simulink model "mrefrobotarm_modified_previous_y_previous_ref"  (R2018b)
settings: Solver=FixedStepAuto  StartTime=0.0  StopTime=60  RelTol=1e-3  AbsTol=1e-6
undefined symbols (not defined in the file or in its folder): sfunxy2
libraries: neural x301, simulink x1
(part 7 of 10)

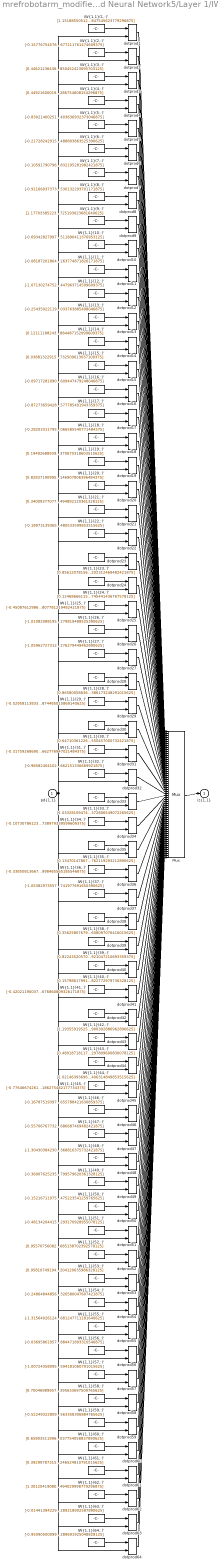
== system mrefrobotarm_modified_previous_y_previous_ref/Feed-Forward Neural Network5/Layer 1/IW{1,1} ==
  "pd{1,1}" : Inport  PortDimensions=8
      mask Display: e = 0.06;c1 = [120 230 180]/255;c2 = ([120 230 180]+0)/(256+128);c3 = ([120 230 180]+128)/(256+128);patch([0 1 1 0],[0 0 1 1],c1);patch([0 1 1 1-e 1-e 0+e],[0 0 1 1-e 0+e 0+e],c2);patch([0 0 1 1-e 0+e 0+e],[0 1 1 1-e 1-e 0+e],c3);plot([0 1 1 0 0],[0 0 1 1 0]);
  "IW{1,1}(1,:)'" : Constant  Value=[1.15188550512719078966483721160329878330230712890625;0.28812102779775983218968349319766275584697723388671875;0.56266210788343784532372637841035611927509307861328125;-0.28333109295564262719580028715427033603191375732421875;0.2157034015099435764195590081726550124585628509521484375;-0.320690714134774623733648013512720353901386260986328125;-1.7558165749549512479887880544993095099925994873046875;-0.445441972828221455227293290590750984847545623779296875]
      mask Display: e = 0.06;c1 = [120 150 230]/255;c2 = ([120 150 230]+0)/383;c3 = ([120 150 230]+128)/383;patch([0 1 1 0],[0 0 1 1],c1);patch([0 1 1 1-e 1-e 0+e],[0 0 1 1-e 0+e 0+e],c2);patch([0 0 1 1-e 0+e 0+e],[0 1 1 1-e 1-e 0+e],c3);plot([0 1 1 0 0],[0 0 1 1 0]);disp('Weights');
  "IW{1,1}(10,:)'" : Constant  Value=[-0.69342827997867140243926087350700981914997100830078125;0.302628053808435326654802111079334281384944915771484375;0.50475756804391236354234706595889292657375335693359375;-0.8382169307464308882771319986204616725444793701171875;0.514118176756543032723811847972683608531951904296875;0.9119975746533526272941116985748521983623504638671875;0.59957744726285355785222463964601047337055206298828125;0.75864381905745237322236107502249069511890411376953125]
      mask Display: e = 0.06;c1 = [120 150 230]/255;c2 = ([120 150 230]+0)/383;c3 = ([120 150 230]+128)/383;patch([0 1 1 0],[0 0 1 1],c1);patch([0 1 1 1-e 1-e 0+e],[0 0 1 1-e 0+e 0+e],c2);patch([0 0 1 1-e 0+e 0+e],[0 1 1 1-e 1-e 0+e],c3);plot([0 1 1 0 0],[0 0 1 1 0]);disp('Weights');
  "IW{1,1}(11,:)'" : Constant  Value=[-0.08187201864334088530217314882975188083946704864501953125;0.73089752966811116774437095955363474786281585693359375;0.5387200520871704423342407608288340270519256591796875;-1.09121606557834116557614834164269268512725830078125;0.9840256530079540819855310473940335214138031005859375;0.413862403720223703817993055054103024303913116455078125;1.027219477112980339228442971943877637386322021484375;-0.66505920483041236490606706865946762263774871826171875]
      mask Display: e = 0.06;c1 = [120 150 230]/255;c2 = ([120 150 230]+0)/383;c3 = ([120 150 230]+128)/383;patch([0 1 1 0],[0 0 1 1],c1);patch([0 1 1 1-e 1-e 0+e],[0 0 1 1-e 0+e 0+e],c2);patch([0 0 1 1-e 0+e 0+e],[0 1 1 1-e 1-e 0+e],c3);plot([0 1 1 0 0],[0 0 1 1 0]);disp('Weights');
  "IW{1,1}(12,:)'" : Constant  Value=[-1.07130274752541776450698307598941028118133544921875;-1.4362522873395537903462582107749767601490020751953125;0.32170080578624327127812421167618595063686370849609375;1.03829812140938404496637303964234888553619384765625;-0.759812891496933762169874171377159655094146728515625;0.602197452374559016874400185770355165004730224609375;0.2151555708852344872550332866012468002736568450927734375;0.328318123712607989883593972990638576447963714599609375]
      mask Display: e = 0.06;c1 = [120 150 230]/255;c2 = ([120 150 230]+0)/383;c3 = ([120 150 230]+128)/383;patch([0 1 1 0],[0 0 1 1],c1);patch([0 1 1 1-e 1-e 0+e],[0 0 1 1-e 0+e 0+e],c2);patch([0 0 1 1-e 0+e 0+e],[0 1 1 1-e 1-e 0+e],c3);plot([0 1 1 0 0],[0 0 1 1 0]);disp('Weights');
  "IW{1,1}(13,:)'" : Constant  Value=[-0.254350221196234016485249185279826633632183074951171875;-1.1795238596441508516221574609517119824886322021484375;0.80833668204856368166844049483188427984714508056640625;0.86038083232116691068114278095890767872333526611328125;-0.450732077477428216827348705919575877487659454345703125;-1.0998838119882419217532287802896462380886077880859375;0.50040120768586004995626126401475630700588226318359375;-0.780004345720864744606615204247646033763885498046875]
      mask Display: e = 0.06;c1 = [120 150 230]/255;c2 = ([120 150 230]+0)/383;c3 = ([120 150 230]+128)/383;patch([0 1 1 0],[0 0 1 1],c1);patch([0 1 1 1-e 1-e 0+e],[0 0 1 1-e 0+e 0+e],c2);patch([0 0 1 1-e 0+e 0+e],[0 1 1 1-e 1-e 0+e],c3);plot([0 1 1 0 0],[0 0 1 1 0]);disp('Weights');
  "IW{1,1}(14,:)'" : Constant  Value=[0.12111188243225030902738836857679416425526142120361328125;1.2254734338665216331065721533377654850482940673828125;-1.2126460475572156116896849198383279144763946533203125;-0.11392876827753649349173059590611956082284450531005859375;0.1615772181693192199869457681415951810777187347412109375;1.061583549738458032152266241610050201416015625;0.10245837646828574729607197468794765882194042205810546875;1.14489655514380839207433382398448884487152099609375]
      mask Display: e = 0.06;c1 = [120 150 230]/255;c2 = ([120 150 230]+0)/383;c3 = ([120 150 230]+128)/383;patch([0 1 1 0],[0 0 1 1],c1);patch([0 1 1 1-e 1-e 0+e],[0 0 1 1-e 0+e 0+e],c2);patch([0 0 1 1-e 0+e 0+e],[0 1 1 1-e 1-e 0+e],c3);plot([0 1 1 0 0],[0 0 1 1 0]);disp('Weights');
  "IW{1,1}(15,:)'" : Constant  Value=[0.038813229156217245174875785096446634270250797271728515625;0.486470279353224788199128170163021422922611236572265625;-0.45894295845177135451109506902866996824741363525390625;0.0276916856546326091426113436000377987511456012725830078125;1.6051967623725589273675495860516093671321868896484375;-0.45590732770331587886403212905861437320709228515625;-0.652539724709438218042123480699956417083740234375;1.0980322803721804802989936433732509613037109375]
      mask Display: e = 0.06;c1 = [120 150 230]/255;c2 = ([120 150 230]+0)/383;c3 = ([120 150 230]+128)/383;patch([0 1 1 0],[0 0 1 1],c1);patch([0 1 1 1-e 1-e 0+e],[0 0 1 1-e 0+e 0+e],c2);patch([0 0 1 1-e 0+e 0+e],[0 1 1 1-e 1-e 0+e],c3);plot([0 1 1 0 0],[0 0 1 1 0]);disp('Weights');
  "IW{1,1}(16,:)'" : Constant  Value=[-0.097172810908892959247395992861129343509674072265625;1.21828113992966802214823474059812724590301513671875;-0.348946678645212615688109281109063886106014251708984375;1.6228867623269358499982217836077325046062469482421875;-0.4468755805697319782865406523342244327068328857421875;0.25552428628844126023977878503501415252685546875;-0.841604705929505758632558354292996227741241455078125;0.384149848353079359508654988530906848609447479248046875]
      mask Display: e = 0.06;c1 = [120 150 230]/255;c2 = ([120 150 230]+0)/383;c3 = ([120 150 230]+128)/383;patch([0 1 1 0],[0 0 1 1],c1);patch([0 1 1 1-e 1-e 0+e],[0 0 1 1-e 0+e 0+e],c2);patch([0 0 1 1-e 0+e 0+e],[0 1 1 1-e 1-e 0+e],c3);plot([0 1 1 0 0],[0 0 1 1 0]);disp('Weights');
  "IW{1,1}(17,:)'" : Constant  Value=[-0.8727365942863782866112387637258507311344146728515625;-1.126434571242459714568440176662988960742950439453125;0.36545685371113723061142763981479220092296600341796875;0.962011466852533470017760919290594756603240966796875;-0.68899715378819259559151078065042383968830108642578125;-0.59210547871686614040953600124339573085308074951171875;-0.06602088688853786913046661766202305443584918975830078125;1.1033314028657768002261718720546923577785491943359375]
      mask Display: e = 0.06;c1 = [120 150 230]/255;c2 = ([120 150 230]+0)/383;c3 = ([120 150 230]+128)/383;patch([0 1 1 0],[0 0 1 1],c1);patch([0 1 1 1-e 1-e 0+e],[0 0 1 1-e 0+e 0+e],c2);patch([0 0 1 1-e 0+e 0+e],[0 1 1 1-e 1-e 0+e],c3);plot([0 1 1 0 0],[0 0 1 1 0]);disp('Weights');
  "IW{1,1}(18,:)'" : Constant  Value=[-0.282033117955742096416571484951418824493885040283203125;-0.09685575267191497139673828087325091473758220672607421875;1.0369904994954521892935872529051266610622406005859375;0.410108416989715340861266668071039021015167236328125;0.5329483580200420345107659159111790359020233154296875;1.0824307275914344383949128314270637929439544677734375;1.0907238106762771057134386865072883665561676025390625;-0.9864564974524812068779056062339805066585540771484375]
      mask Display: e = 0.06;c1 = [120 150 230]/255;c2 = ([120 150 230]+0)/383;c3 = ([120 150 230]+128)/383;patch([0 1 1 0],[0 0 1 1],c1);patch([0 1 1 1-e 1-e 0+e],[0 0 1 1-e 0+e 0+e],c2);patch([0 0 1 1-e 0+e 0+e],[0 1 1 1-e 1-e 0+e],c3);plot([0 1 1 0 0],[0 0 1 1 0]);disp('Weights');
  "IW{1,1}(19,:)'" : Constant  Value=[0.19492688939710911544267446515732444822788238525390625;0.28850729483225101557053449141676537692546844482421875;-0.175773740393380395463651666432269848883152008056640625;-1.89756443554498854808798569138161838054656982421875;-0.5054315086265079859373372528352774679660797119140625;1.0667368662509619792189141662674956023693084716796875;0.19891400645817736148046606103889644145965576171875;0.567362684381534254640655490220524370670318603515625]
      mask Display: e = 0.06;c1 = [120 150 230]/255;c2 = ([120 150 230]+0)/383;c3 = ([120 150 230]+128)/383;patch([0 1 1 0],[0 0 1 1],c1);patch([0 1 1 1-e 1-e 0+e],[0 0 1 1-e 0+e 0+e],c2);patch([0 0 1 1-e 0+e 0+e],[0 1 1 1-e 1-e 0+e],c3);plot([0 1 1 0 0],[0 0 1 1 0]);disp('Weights');
  "IW{1,1}(2,:)'" : Constant  Value=[-0.15776754576942597640965004757163114845752716064453125;-0.455993213383465434418440054287202656269073486328125;1.1839932390166734155201311295968480408191680908203125;0.29937087607287893309404580577393062412738800048828125;-0.0048999116352581063849047637859257520176470279693603515625;0.049281318949005371854443779966459260322153568267822265625;-1.1301308079633043401912573244771920144557952880859375;-1.494209820076525030430047991103492677211761474609375]
      mask Display: e = 0.06;c1 = [120 150 230]/255;c2 = ([120 150 230]+0)/383;c3 = ([120 150 230]+128)/383;patch([0 1 1 0],[0 0 1 1],c1);patch([0 1 1 1-e 1-e 0+e],[0 0 1 1-e 0+e 0+e],c2);patch([0 0 1 1-e 0+e 0+e],[0 1 1 1-e 1-e 0+e],c3);plot([0 1 1 0 0],[0 0 1 1 0]);disp('Weights');
  "IW{1,1}(20,:)'" : Constant  Value=[0.8283719099560700183104700045078061521053314208984375;-0.9420385849900030361681046997546218335628509521484375;0.83950886137076008441937347015482373535633087158203125;-0.94073002472129407802725609144545160233974456787109375;-0.58905367954073117875424259182182140648365020751953125;0.9613658421825383992853630843455903232097625732421875;0.6352455319925611743059334912686608731746673583984375;0.551159922915347433303168145357631146907806396484375]
      mask Display: e = 0.06;c1 = [120 150 230]/255;c2 = ([120 150 230]+0)/383;c3 = ([120 150 230]+128)/383;patch([0 1 1 0],[0 0 1 1],c1);patch([0 1 1 1-e 1-e 0+e],[0 0 1 1-e 0+e 0+e],c2);patch([0 0 1 1-e 0+e 0+e],[0 1 1 1-e 1-e 0+e],c3);plot([0 1 1 0 0],[0 0 1 1 0]);disp('Weights');
  "IW{1,1}(21,:)'" : Constant  Value=[0.34009377077838232050766009706421755254268646240234375;-0.466780497991363285681387651493423618376255035400390625;1.2292709966424573142518283930257894098758697509765625;-0.88137293354350243479444770855479873716831207275390625;-0.7761093614509670945977859446429647505283355712890625;-0.160844472776546176806533594572101719677448272705078125;0.9128574666560584915941944927908480167388916015625;-1.0472251078619354558441045810468494892120361328125]
      mask Display: e = 0.06;c1 = [120 150 230]/255;c2 = ([120 150 230]+0)/383;c3 = ([120 150 230]+128)/383;patch([0 1 1 0],[0 0 1 1],c1);patch([0 1 1 1-e 1-e 0+e],[0 0 1 1-e 0+e 0+e],c2);patch([0 0 1 1-e 0+e 0+e],[0 1 1 1-e 1-e 0+e],c3);plot([0 1 1 0 0],[0 0 1 1 0]);disp('Weights');
  "IW{1,1}(22,:)'" : Constant  Value=[-0.189731393651665081190316186621203087270259857177734375;-0.72495794035112359754435829017893411219120025634765625;0.9357984514248178786743892487720586359500885009765625;-1.0869305870717254070001445143134333193302154541015625;-0.50973886964233405816315780612058006227016448974609375;0.473915859680547002508177456547855399549007415771484375;1.0230173709565664186271760627278126776218414306640625;0.9914709747258270144953939961851574480533599853515625]
      mask Display: e = 0.06;c1 = [120 150 230]/255;c2 = ([120 150 230]+0)/383;c3 = ([120 150 230]+128)/383;patch([0 1 1 0],[0 0 1 1],c1);patch([0 1 1 1-e 1-e 0+e],[0 0 1 1-e 0+e 0+e],c2);patch([0 0 1 1-e 0+e 0+e],[0 1 1 1-e 1-e 0+e],c3);plot([0 1 1 0 0],[0 0 1 1 0]);disp('Weights');
  "IW{1,1}(23,:)'" : Constant  Value=[0.856120781560206989269090627203695476055145263671875;-1.069464124720405973079095929278992116451263427734375;0.2919731447302797988641032134182751178741455078125;0.6061622306072764754247828022926114499568939208984375;-0.653691930601032478165279826498590409755706787109375;-0.88804792534942789128393769715330563485622406005859375;-1.0119635839619267603239904929068870842456817626953125;0.95988282102991540067904452371294610202312469482421875]
      mask Display: e = 0.06;c1 = [120 150 230]/255;c2 = ([120 150 230]+0)/383;c3 = ([120 150 230]+128)/383;patch([0 1 1 0],[0 0 1 1],c1);patch([0 1 1 1-e 1-e 0+e],[0 0 1 1-e 0+e 0+e],c2);patch([0 0 1 1-e 0+e 0+e],[0 1 1 1-e 1-e 0+e],c3);plot([0 1 1 0 0],[0 0 1 1 0]);disp('Weights');
  "IW{1,1}(24,:)'" : Constant  Value=[0.124686661157710043656976495185517705976963043212890625;-0.8210810741082565922255298573873005807399749755859375;1.1767856627094956945001058556954376399517059326171875;0.1691193234330329586700969457524479366838932037353515625;-1.12605095295487611650742110214196145534515380859375;-0.96214809238136800306762097534374333918094635009765625;-0.95747311663602430176212010337621904909610748291015625;-0.8403367277084676789655759421293623745441436767578125]
      mask Display: e = 0.06;c1 = [120 150 230]/255;c2 = ([120 150 230]+0)/383;c3 = ([120 150 230]+128)/383;patch([0 1 1 0],[0 0 1 1],c1);patch([0 1 1 1-e 1-e 0+e],[0 0 1 1-e 0+e 0+e],c2);patch([0 0 1 1-e 0+e 0+e],[0 1 1 1-e 1-e 0+e],c3);plot([0 1 1 0 0],[0 0 1 1 0]);disp('Weights');
  "IW{1,1}(25,:)'" : Constant  Value=[-0.4508761298608821022071424522437155246734619140625;1.0106688771579630525820903130806982517242431640625;-0.1774785669335633697674126096899271942675113677978515625;0.488867822831043519204996528060291893780231475830078125;-0.523769084982353749779804275021888315677642822265625;0.5469050128236101482315234534326009452342987060546875;1.628688158073976932627147107268683612346649169921875;0.2267927559895878963924786830830271355807781219482421875]
      mask Display: e = 0.06;c1 = [120 150 230]/255;c2 = ([120 150 230]+0)/383;c3 = ([120 150 230]+128)/383;patch([0 1 1 0],[0 0 1 1],c1);patch([0 1 1 1-e 1-e 0+e],[0 0 1 1-e 0+e 0+e],c2);patch([0 0 1 1-e 0+e 0+e],[0 1 1 1-e 1-e 0+e],c3);plot([0 1 1 0 0],[0 0 1 1 0]);disp('Weights');
  "IW{1,1}(26,:)'" : Constant  Value=[-1.01082088195786301554335295804776251316070556640625;0.95465379283400275678417301605804823338985443115234375;0.391386386609228142940963834917056374251842498779296875;1.4225990849750778100002435166970826685428619384765625;-0.73545495103985902840548760650563053786754608154296875;-0.736133991802305320817367828567512333393096923828125;0.442114848390933234956179376240470446646213531494140625;0.43657172644220987312024817583733238279819488525390625]
      mask Display: e = 0.06;c1 = [120 150 230]/255;c2 = ([120 150 230]+0)/383;c3 = ([120 150 230]+128)/383;patch([0 1 1 0],[0 0 1 1],c1);patch([0 1 1 1-e 1-e 0+e],[0 0 1 1-e 0+e 0+e],c2);patch([0 0 1 1-e 0+e 0+e],[0 1 1 1-e 1-e 0+e],c3);plot([0 1 1 0 0],[0 0 1 1 0]);disp('Weights');
  "IW{1,1}(27,:)'" : Constant  Value=[-1.0596272731227285301969232023111544549465179443359375;-0.54530840839943228726127699701464734971523284912109375;0.6278313816556941873159303213469684123992919921875;0.270771156859894279733680377830751240253448486328125;0.464390599696782147010054586644400842487812042236328125;-0.53372241047857371665230630242149345576763153076171875;0.956306487503788549275896002654917538166046142578125;1.47074764980775629652498537325300276279449462890625]
      mask Display: e = 0.06;c1 = [120 150 230]/255;c2 = ([120 150 230]+0)/383;c3 = ([120 150 230]+128)/383;patch([0 1 1 0],[0 0 1 1],c1);patch([0 1 1 1-e 1-e 0+e],[0 0 1 1-e 0+e 0+e],c2);patch([0 0 1 1-e 0+e 0+e],[0 1 1 1-e 1-e 0+e],c3);plot([0 1 1 0 0],[0 0 1 1 0]);disp('Weights');
  "IW{1,1}(28,:)'" : Constant  Value=[0.86580058636540346839183257543481886386871337890625;0.9756419600736609964997114730067551136016845703125;-1.2316073907028701750476784582133404910564422607421875;-1.03033429662976772078764042817056179046630859375;0.1339502814816569686851011056205607019364833831787109375;0.74929830934803554054468577305669896304607391357421875;0.0743680662885670973327734145641443319618701934814453125;-0.80516734717865345860587922288686968386173248291015625]
      mask Display: e = 0.06;c1 = [120 150 230]/255;c2 = ([120 150 230]+0)/383;c3 = ([120 150 230]+128)/383;patch([0 1 1 0],[0 0 1 1],c1);patch([0 1 1 1-e 1-e 0+e],[0 0 1 1-e 0+e 0+e],c2);patch([0 0 1 1-e 0+e 0+e],[0 1 1 1-e 1-e 0+e],c3);plot([0 1 1 0 0],[0 0 1 1 0]);disp('Weights');
  "IW{1,1}(29,:)'" : Constant  Value=[-0.5295811383351869405800016465946100652217864990234375;-0.278717330509984650976917919251718558371067047119140625;-0.66606714661326493764903489136486314237117767333984375;-0.8798401281044869737257840824895538389682769775390625;0.268788230217950785405633951086201705038547515869140625;-1.5135879192232033485510100945248268544673919677734375;0.91318255242783175074094970113947056233882904052734375;0.920699349371988606804961818852461874485015869140625]
      mask Display: e = 0.06;c1 = [120 150 230]/255;c2 = ([120 150 230]+0)/383;c3 = ([120 150 230]+128)/383;patch([0 1 1 0],[0 0 1 1],c1);patch([0 1 1 1-e 1-e 0+e],[0 0 1 1-e 0+e 0+e],c2);patch([0 0 1 1-e 0+e 0+e],[0 1 1 1-e 1-e 0+e],c3);plot([0 1 1 0 0],[0 0 1 1 0]);disp('Weights');
  "IW{1,1}(3,:)'" : Constant  Value=[0.446212364360280389075086304728756658732891082763671875;-0.0978189681976021907505725039300159551203250885009765625;-1.31393838489276415515405460610054433345794677734375;-0.79167290442859183929869004714419133961200714111328125;1.1377022565084218275188732150127179920673370361328125;0.0090609210361883817108630267966873361729085445404052734375;-1.231014577077934379900625572190620005130767822265625;-0.1951198768884519207933436746316147036850452423095703125]
      mask Display: e = 0.06;c1 = [120 150 230]/255;c2 = ([120 150 230]+0)/383;c3 = ([120 150 230]+128)/383;patch([0 1 1 0],[0 0 1 1],c1);patch([0 1 1 1-e 1-e 0+e],[0 0 1 1-e 0+e 0+e],c2);patch([0 0 1 1-e 0+e 0+e],[0 1 1 1-e 1-e 0+e],c3);plot([0 1 1 0 0],[0 0 1 1 0]);disp('Weights');
  "IW{1,1}(30,:)'" : Constant  Value=[0.6471036122667062073787747067399322986602783203125;-0.061940615906763842046789392270511598326265811920166015625;-0.312052580594836259653135357439168728888034820556640625;1.2990947753306822942676035381737165153026580810546875;-0.0036105482406158756307490431680662368307821452617645263671875;-0.42311702194302835966510656362515874207019805908203125;0.88830861509092995387248947736225090920925140380859375;-1.6478565407139675880188178780372254550457000732421875]
      mask Display: e = 0.06;c1 = [120 150 230]/255;c2 = ([120 150 230]+0)/383;c3 = ([120 150 230]+128)/383;patch([0 1 1 0],[0 0 1 1],c1);patch([0 1 1 1-e 1-e 0+e],[0 0 1 1-e 0+e 0+e],c2);patch([0 0 1 1-e 0+e 0+e],[0 1 1 1-e 1-e 0+e],c3);plot([0 1 1 0 0],[0 0 1 1 0]);disp('Weights');
  "IW{1,1}(31,:)'" : Constant  Value=[-0.31759268690855346761736655025742948055267333984375;-0.4042457377349506497665743154357187449932098388671875;0.251357110918958459588878895374364219605922698974609375;-1.10791367956164332753132839570753276348114013671875;0.73836626855680165260054081954876892268657684326171875;1.032559094167967206345792874344624578952789306640625;-1.070606342674453426155878332792781293392181396484375;1.126008088640405357949703102349303662776947021484375]
      mask Display: e = 0.06;c1 = [120 150 230]/255;c2 = ([120 150 230]+0)/383;c3 = ([120 150 230]+128)/383;patch([0 1 1 0],[0 0 1 1],c1);patch([0 1 1 1-e 1-e 0+e],[0 0 1 1-e 0+e 0+e],c2);patch([0 0 1 1-e 0+e 0+e],[0 1 1 1-e 1-e 0+e],c3);plot([0 1 1 0 0],[0 0 1 1 0]);disp('Weights');
  "IW{1,1}(32,:)'" : Constant  Value=[-0.98582404102823650848819170278147794306278228759765625;0.110955204356297743029102775835781358182430267333984375;1.1171545662955260080906327857519499957561492919921875;-0.086582673998257642100639941418194212019443511962890625;1.0183086056376919881216736030182801187038421630859375;-0.146176428296484084423667582086636684834957122802734375;-1.27212378176424056874793677707202732563018798828125;0.778085451655250448510514615918509662151336669921875]
      mask Display: e = 0.06;c1 = [120 150 230]/255;c2 = ([120 150 230]+0)/383;c3 = ([120 150 230]+128)/383;patch([0 1 1 0],[0 0 1 1],c1);patch([0 1 1 1-e 1-e 0+e],[0 0 1 1-e 0+e 0+e],c2);patch([0 0 1 1-e 0+e 0+e],[0 1 1 1-e 1-e 0+e],c3);plot([0 1 1 0 0],[0 0 1 1 0]);disp('Weights');
  "IW{1,1}(33,:)'" : Constant  Value=[1.0332810947416766200745996684418059885501861572265625;1.1881751882562401334553214837796986103057861328125;0.0113711764073888312032156733266674564220011234283447265625;0.54613530436783752630702792885131202638149261474609375;0.8575124714924264868187719912384636700153350830078125;-0.9807149901858362994744311436079442501068115234375;-0.08504032072985522050512230407548486255109310150146484375;-0.86010602226781662782428838909254409372806549072265625]
      mask Display: e = 0.06;c1 = [120 150 230]/255;c2 = ([120 150 230]+0)/383;c3 = ([120 150 230]+128)/383;patch([0 1 1 0],[0 0 1 1],c1);patch([0 1 1 1-e 1-e 0+e],[0 0 1 1-e 0+e 0+e],c2);patch([0 0 1 1-e 0+e 0+e],[0 1 1 1-e 1-e 0+e],c3);plot([0 1 1 0 0],[0 0 1 1 0]);disp('Weights');
  "IW{1,1}(34,:)'" : Constant  Value=[-0.10730786123257247954843052184514817781746387481689453125;-1.2561740133845915590171671283314935863018035888671875;0.1916023081249165205264262112905271351337432861328125;-0.733724466418752552243631726014427840709686279296875;-1.19798795607447328137595832231454551219940185546875;0.395299789476157126255628782018902711570262908935546875;1.2942966424689743565323851726134307682514190673828125;0.2851043720773309697591457734233699738979339599609375]
      mask Display: e = 0.06;c1 = [120 150 230]/255;c2 = ([120 150 230]+0)/383;c3 = ([120 150 230]+128)/383;patch([0 1 1 0],[0 0 1 1],c1);patch([0 1 1 1-e 1-e 0+e],[0 0 1 1-e 0+e 0+e],c2);patch([0 0 1 1-e 0+e 0+e],[0 1 1 1-e 1-e 0+e],c3);plot([0 1 1 0 0],[0 0 1 1 0]);disp('Weights');
  "IW{1,1}(35,:)'" : Constant  Value=[0.13470147867077508774258376433863304555416107177734375;0.89180318892628818172596538715879432857036590576171875;-1.251923878018734281880597336567007005214691162109375;1.0584028339053215272969055149587802588939666748046875;-0.466690066426573457736282080077216960489749908447265625;0.80408658190793047548794447720865719020366668701171875;0.80069797512159424091038317783386446535587310791015625;0.65001316148328280863921690979623235762119293212890625]
      mask Display: e = 0.06;c1 = [120 150 230]/255;c2 = ([120 150 230]+0)/383;c3 = ([120 150 230]+128)/383;patch([0 1 1 0],[0 0 1 1],c1);patch([0 1 1 1-e 1-e 0+e],[0 0 1 1-e 0+e 0+e],c2);patch([0 0 1 1-e 0+e 0+e],[0 1 1 1-e 1-e 0+e],c3);plot([0 1 1 0 0],[0 0 1 1 0]);disp('Weights');
  "IW{1,1}(36,:)'" : Constant  Value=[-0.3385081366785949175124414978199638426303863525390625;-0.69503528690295102165919161052443087100982666015625;0.4923281094682134817475116506102494895458221435546875;-0.720964622145814804099472894449718296527862548828125;-0.2556243474584316555109353430452756583690643310546875;-1.1219523070902417405392270666197873651981353759765625;-1.060868790922331328374639269895851612091064453125;-1.28292959603458012196597337606362998485565185546875]
      mask Display: e = 0.06;c1 = [120 150 230]/255;c2 = ([120 150 230]+0)/383;c3 = ([120 150 230]+128)/383;patch([0 1 1 0],[0 0 1 1],c1);patch([0 1 1 1-e 1-e 0+e],[0 0 1 1-e 0+e 0+e],c2);patch([0 0 1 1-e 0+e 0+e],[0 1 1 1-e 1-e 0+e],c3);plot([0 1 1 0 0],[0 0 1 1 0]);disp('Weights');
  "IW{1,1}(37,:)'" : Constant  Value=[-1.0538297355717778369665893478668294847011566162109375;0.9137438889102564854027832552674226462841033935546875;0.330465292020934608974158663841080851852893829345703125;-0.469046635263795697046163013510522432625293731689453125;0.76983143635499262646959550693281926214694976806640625;1.2274381452821707672029560853843577206134796142578125;-0.9594647793827260073840079712681472301483154296875;0.4807491192598087881293622558587230741977691650390625]
      mask Display: e = 0.06;c1 = [120 150 230]/255;c2 = ([120 150 230]+0)/383;c3 = ([120 150 230]+128)/383;patch([0 1 1 0],[0 0 1 1],c1);patch([0 1 1 1-e 1-e 0+e],[0 0 1 1-e 0+e 0+e],c2);patch([0 0 1 1-e 0+e 0+e],[0 1 1 1-e 1-e 0+e],c3);plot([0 1 1 0 0],[0 0 1 1 0]);disp('Weights');
  "IW{1,1}(38,:)'" : Constant  Value=[0.35625807679689269757972169827553443610668182373046875;0.1331977864564148072989979709745966829359531402587890625;-0.365682952283444662189282325925887562334537506103515625;-1.0953170441072181962027798363124020397663116455078125;0.8305354135097473555759961527655832469463348388671875;1.085738228001417837731423787772655487060546875;1.0659017284151206528264310691156424582004547119140625;0.807218132587677050793217858881689608097076416015625]
      mask Display: e = 0.06;c1 = [120 150 230]/255;c2 = ([120 150 230]+0)/383;c3 = ([120 150 230]+128)/383;patch([0 1 1 0],[0 0 1 1],c1);patch([0 1 1 1-e 1-e 0+e],[0 0 1 1-e 0+e 0+e],c2);patch([0 0 1 1-e 0+e 0+e],[0 1 1 1-e 1-e 0+e],c3);plot([0 1 1 0 0],[0 0 1 1 0]);disp('Weights');
  "IW{1,1}(39,:)'" : Constant  Value=[0.82243520570661321489325246147927828133106231689453125;-0.92744873138334449347297550048097036778926849365234375;-0.5659382507761587799421931777033023536205291748046875;1.10287668857012288725627513485960662364959716796875;0.6500558112044181324762348594958893954753875732421875;-0.279365585293477491912739196777692995965480804443359375;-0.329420056930422811003467131740762852132320404052734375;1.214469321330822193516496554366312921047210693359375]
      mask Display: e = 0.06;c1 = [120 150 230]/255;c2 = ([120 150 230]+0)/383;c3 = ([120 150 230]+128)/383;patch([0 1 1 0],[0 0 1 1],c1);patch([0 1 1 1-e 1-e 0+e],[0 0 1 1-e 0+e 0+e],c2);patch([0 0 1 1-e 0+e 0+e],[0 1 1 1-e 1-e 0+e],c3);plot([0 1 1 0 0],[0 0 1 1 0]);disp('Weights');
  "IW{1,1}(4,:)'" : Constant  Value=[0.449216000193385534000611869487329386174678802490234375;1.069092416755129004712898677098564803600311279296875;1.1202529630482478406605650889105163514614105224609375;0.88723055542406170648206398254842497408390045166015625;-0.53693856516414084634192249723128043115139007568359375;-0.8953535921229356375761199160479009151458740234375;-0.424853262852135316052226698957383632659912109375;0.98558770378236093545609719512867741286754608154296875]
      mask Display: e = 0.06;c1 = [120 150 230]/255;c2 = ([120 150 230]+0)/383;c3 = ([120 150 230]+128)/383;patch([0 1 1 0],[0 0 1 1],c1);patch([0 1 1 1-e 1-e 0+e],[0 0 1 1-e 0+e 0+e],c2);patch([0 0 1 1-e 0+e 0+e],[0 1 1 1-e 1-e 0+e],c3);plot([0 1 1 0 0],[0 0 1 1 0]);disp('Weights');
  "IW{1,1}(40,:)'" : Constant  Value=[0.1579861799126709431817516815499402582645416259765625;0.2440200417363912188672969705294235609471797943115234375;-1.254796483799876849474230766645632684230804443359375;0.5053076788989432355236885996419005095958709716796875;0.050687802700905726371871651281253434717655181884765625;1.485676910567629960269186994992196559906005859375;-0.4868889044458868387010852529783733189105987548828125;0.86657970142906493027368242110242135822772979736328125]
      mask Display: e = 0.06;c1 = [120 150 230]/255;c2 = ([120 150 230]+0)/383;c3 = ([120 150 230]+128)/383;patch([0 1 1 0],[0 0 1 1],c1);patch([0 1 1 1-e 1-e 0+e],[0 0 1 1-e 0+e 0+e],c2);patch([0 0 1 1-e 0+e 0+e],[0 1 1 1-e 1-e 0+e],c3);plot([0 1 1 0 0],[0 0 1 1 0]);disp('Weights');
  "IW{1,1}(41,:)'" : Constant  Value=[-0.420211900371094182471409794743522070348262786865234375;-0.27063223612642517412751885785837657749652862548828125;-1.3818974261721799212665473532979376614093780517578125;0.439043108327200837237569430726580321788787841796875;0.252756123195656379198936747343395836651325225830078125;0.9748376953007487077940140807186253368854522705078125;1.301748762070959575254391893395222723484039306640625;-0.258835755420718793828882553498260676860809326171875]
      mask Display: e = 0.06;c1 = [120 150 230]/255;c2 = ([120 150 230]+0)/383;c3 = ([120 150 230]+128)/383;patch([0 1 1 0],[0 0 1 1],c1);patch([0 1 1 1-e 1-e 0+e],[0 0 1 1-e 0+e 0+e],c2);patch([0 0 1 1-e 0+e 0+e],[0 1 1 1-e 1-e 0+e],c3);plot([0 1 1 0 0],[0 0 1 1 0]);disp('Weights');
  "IW{1,1}(42,:)'" : Constant  Value=[1.1935591952557018657898879610002040863037109375;-0.71105824460165323319671415447373874485492706298828125;-0.7263367042612871582463185404776595532894134521484375;-0.63193248648512756471262719060177914798259735107421875;-0.491876962907790982182376637865672819316387176513671875;-0.711285782067984317933451166027225553989410400390625;1.139204332500781902126618660986423492431640625;-0.48345043676651366926222408437752164900302886962890625]
      mask Display: e = 0.06;c1 = [120 150 230]/255;c2 = ([120 150 230]+0)/383;c3 = ([120 150 230]+128)/383;patch([0 1 1 0],[0 0 1 1],c1);patch([0 1 1 1-e 1-e 0+e],[0 0 1 1-e 0+e 0+e],c2);patch([0 0 1 1-e 0+e 0+e],[0 1 1 1-e 1-e 0+e],c3);plot([0 1 1 0 0],[0 0 1 1 0]);disp('Weights');
  "IW{1,1}(43,:)'" : Constant  Value=[0.489187181174163432384460747925913892686367034912109375;0.477596097486275461552196475167875178158283233642578125;-0.795458358727680892030775794410146772861480712890625;-0.434416995971317498881347773931338451802730560302734375;1.380919483840138628494287331704981625080108642578125;1.3794778054486453999771811140817590057849884033203125;-0.0945329309601852241229380524600856006145477294921875;0.297361684400176351505962202281807549297809600830078125]
      mask Display: e = 0.06;c1 = [120 150 230]/255;c2 = ([120 150 230]+0)/383;c3 = ([120 150 230]+128)/383;patch([0 1 1 0],[0 0 1 1],c1);patch([0 1 1 1-e 1-e 0+e],[0 0 1 1-e 0+e 0+e],c2);patch([0 0 1 1-e 0+e 0+e],[0 1 1 1-e 1-e 0+e],c3);plot([0 1 1 0 0],[0 0 1 1 0]);disp('Weights');
  "IW{1,1}(44,:)'" : Constant  Value=[1.0214639369626332676688207357074134051799774169921875;-0.9535830397905560307236783046391792595386505126953125;-1.0500790082631608068908235509297810494899749755859375;-0.1813927349484561191150788772574742324650287628173828125;-1.1748803936902361133576278007240034639835357666015625;0.76731553335516300418106538927531801164150238037109375;-0.0912843346818332512793148225682671181857585906982421875;0.4658321414014621186794329332769848406314849853515625]
      mask Display: e = 0.06;c1 = [120 150 230]/255;c2 = ([120 150 230]+0)/383;c3 = ([120 150 230]+128)/383;patch([0 1 1 0],[0 0 1 1],c1);patch([0 1 1 1-e 1-e 0+e],[0 0 1 1-e 0+e 0+e],c2);patch([0 0 1 1-e 0+e 0+e],[0 1 1 1-e 1-e 0+e],c3);plot([0 1 1 0 0],[0 0 1 1 0]);disp('Weights');
  "IW{1,1}(45,:)'" : Constant  Value=[-0.77646674261790382676196031752624548971652984619140625;1.3904720272430639571581423297175206243991851806640625;0.2135474215962842314819880584764177910983562469482421875;0.343795791976723441596419661436812020838260650634765625;-0.66963107464097959553583905289997346699237823486328125;-1.135393046063842614756822513299994170665740966796875;0.5568997405401947542458174211787991225719451904296875;-0.6827481520692850747167312874807976186275482177734375]
      mask Display: e = 0.06;c1 = [120 150 230]/255;c2 = ([120 150 230]+0)/383;c3 = ([120 150 230]+128)/383;patch([0 1 1 0],[0 0 1 1],c1);patch([0 1 1 1-e 1-e 0+e],[0 0 1 1-e 0+e 0+e],c2);patch([0 0 1 1-e 0+e 0+e],[0 1 1 1-e 1-e 0+e],c3);plot([0 1 1 0 0],[0 0 1 1 0]);disp('Weights');
  "IW{1,1}(46,:)'" : Constant  Value=[-0.167875193971138203519188891732483170926570892333984375;-0.439229024609157636671596947053330950438976287841796875;-0.62157862570253052947322203181101940572261810302734375;1.0952847248913843980488991292077116668224334716796875;0.21702485414310157540995760427904315292835235595703125;-0.9358929081924483028842587373219430446624755859375;1.15860580212642094721786634181626141071319580078125;-1.2276578316823429926074595641694031655788421630859375]
      mask Display: e = 0.06;c1 = [120 150 230]/255;c2 = ([120 150 230]+0)/383;c3 = ([120 150 230]+128)/383;patch([0 1 1 0],[0 0 1 1],c1);patch([0 1 1 1-e 1-e 0+e],[0 0 1 1-e 0+e 0+e],c2);patch([0 0 1 1-e 0+e 0+e],[0 1 1 1-e 1-e 0+e],c3);plot([0 1 1 0 0],[0 0 1 1 0]);disp('Weights');
  "IW{1,1}(47,:)'" : Constant  Value=[-0.55706767732511408564022303835372440516948699951171875;-0.72517378784069197461548128558206371963024139404296875;0.494343466819654298038955175798037089407444000244140625;-0.95039953083350836582354759229929186403751373291015625;0.94113936003819975706363720746594481170177459716796875;0.5599009502379292957385814588633365929126739501953125;0.8801931344246025634703300966066308319568634033203125;1.0056252940372996107498693163506686687469482421875]
      mask Display: e = 0.06;c1 = [120 150 230]/255;c2 = ([120 150 230]+0)/383;c3 = ([120 150 230]+128)/383;patch([0 1 1 0],[0 0 1 1],c1);patch([0 1 1 1-e 1-e 0+e],[0 0 1 1-e 0+e 0+e],c2);patch([0 0 1 1-e 0+e 0+e],[0 1 1 1-e 1-e 0+e],c3);plot([0 1 1 0 0],[0 0 1 1 0]);disp('Weights');
  "IW{1,1}(48,:)'" : Constant  Value=[-1.3043038423078154863787858630530536174774169921875;-0.63690338779938249214040979495621286332607269287109375;1.1277002952469936669643857385381124913692474365234375;0.53179836080302045342449446252430789172649383544921875;-0.149019493553352422310354086221195757389068603515625;1.0465617010250920504432770030689425766468048095703125;-0.30508000967842152650888465359457768499851226806640625;-0.74925458817025336610839758577640168368816375732421875]
      mask Display: e = 0.06;c1 = [120 150 230]/255;c2 = ([120 150 230]+0)/383;c3 = ([120 150 230]+128)/383;patch([0 1 1 0],[0 0 1 1],c1);patch([0 1 1 1-e 1-e 0+e],[0 0 1 1-e 0+e 0+e],c2);patch([0 0 1 1-e 0+e 0+e],[0 1 1 1-e 1-e 0+e],c3);plot([0 1 1 0 0],[0 0 1 1 0]);disp('Weights');
  "IW{1,1}(49,:)'" : Constant  Value=[-0.3600762523565881334519644951797090470790863037109375;-0.498905020252015496406983174892957322299480438232421875;-1.404265996561349094662318748305551707744598388671875;1.6043843858166824123401283941348083317279815673828125;0.70962727623678911736959662448498420417308807373046875;0.65612601453902519299532514196471311151981353759765625;0.125251384093528594920741170426481403410434722900390625;-0.026169839130893053635862344208362628705799579620361328125]
      mask Display: e = 0.06;c1 = [120 150 230]/255;c2 = ([120 150 230]+0)/383;c3 = ([120 150 230]+128)/383;patch([0 1 1 0],[0 0 1 1],c1);patch([0 1 1 1-e 1-e 0+e],[0 0 1 1-e 0+e 0+e],c2);patch([0 0 1 1-e 0+e 0+e],[0 1 1 1-e 1-e 0+e],c3);plot([0 1 1 0 0],[0 0 1 1 0]);disp('Weights');
  "IW{1,1}(5,:)'" : Constant  Value=[-0.8302140025142044077455238948459737002849578857421875;-0.99126051208972121298046431547845713794231414794921875;-0.49924369273723556705846249315072782337665557861328125;1.0344687526481990413884659574250690639019012451171875;0.24945181990289888585010658061946742236614227294921875;-1.35430880805712394732154280063696205615997314453125;0.77612575586711918251836550552980042994022369384765625;0.2276343582412316546292885277580353431403636932373046875]
      mask Display: e = 0.06;c1 = [120 150 230]/255;c2 = ([120 150 230]+0)/383;c3 = ([120 150 230]+128)/383;patch([0 1 1 0],[0 0 1 1],c1);patch([0 1 1 1-e 1-e 0+e],[0 0 1 1-e 0+e 0+e],c2);patch([0 0 1 1-e 0+e 0+e],[0 1 1 1-e 1-e 0+e],c3);plot([0 1 1 0 0],[0 0 1 1 0]);disp('Weights');
  "IW{1,1}(50,:)'" : Constant  Value=[-0.152167119759484048557851565419696271419525146484375;1.412190507885614731975465474533848464488983154296875;-1.01574035720856148401480822940357029438018798828125;-0.372612898382188195700592814318952150642871856689453125;1.5063788648286291493860744594712741672992706298828125;0.0527906580427834615232285386809962801635265350341796875;-0.2687976797083513336161786355660296976566314697265625;0.180584806700717470651085250210599042475223541259765625]
      mask Display: e = 0.06;c1 = [120 150 230]/255;c2 = ([120 150 230]+0)/383;c3 = ([120 150 230]+128)/383;patch([0 1 1 0],[0 0 1 1],c1);patch([0 1 1 1-e 1-e 0+e],[0 0 1 1-e 0+e 0+e],c2);patch([0 0 1 1-e 0+e 0+e],[0 1 1 1-e 1-e 0+e],c3);plot([0 1 1 0 0],[0 0 1 1 0]);disp('Weights');
  "IW{1,1}(51,:)'" : Constant  Value=[-0.481342044152840597970310909659019671380519866943359375;0.7167093283518024549039182602427899837493896484375;1.0208102725817476130742988971178419888019561767578125;1.1586595390145928430314370416454039514064788818359375;-0.67658162140217148472487451726919971406459808349609375;-1.190892973127208431805001964676193892955780029296875;0.92724595203779169860780484668794088065624237060546875;0.11810658925822999087973386167504941113293170928955078125]
      mask Display: e = 0.06;c1 = [120 150 230]/255;c2 = ([120 150 230]+0)/383;c3 = ([120 150 230]+128)/383;patch([0 1 1 0],[0 0 1 1],c1);patch([0 1 1 1-e 1-e 0+e],[0 0 1 1-e 0+e 0+e],c2);patch([0 0 1 1-e 0+e 0+e],[0 1 1 1-e 1-e 0+e],c3);plot([0 1 1 0 0],[0 0 1 1 0]);disp('Weights');
  "IW{1,1}(52,:)'" : Constant  Value=[0.9557075608294212099025344286928884685039520263671875;-1.2326721492611711905595939242630265653133392333984375;0.54949090747148610081040942532126791775226593017578125;0.316245885266282888981237420011893846094608306884765625;0.628546150828634520024706944241188466548919677734375;0.0034270941188005942489025468233876381418667733669281005859375;-0.606384787905841715627275334554724395275115966796875;0.98923534671398194451086283152108080685138702392578125]
      mask Display: e = 0.06;c1 = [120 150 230]/255;c2 = ([120 150 230]+0)/383;c3 = ([120 150 230]+128)/383;patch([0 1 1 0],[0 0 1 1],c1);patch([0 1 1 1-e 1-e 0+e],[0 0 1 1-e 0+e 0+e],c2);patch([0 0 1 1-e 0+e 0+e],[0 1 1 1-e 1-e 0+e],c3);plot([0 1 1 0 0],[0 0 1 1 0]);disp('Weights');
  "IW{1,1}(53,:)'" : Constant  Value=[0.9581074919459025007739683132967911660671234130859375;-0.5521564573722728130888981468160636723041534423828125;1.198604056222848601720443184603936970233917236328125;0.87918300593945752918756397775723598897457122802734375;-0.8187774282508166745486732907011173665523529052734375;0.7450409343441080078918048457126133143901824951171875;-0.61911190889374034806991176083101890981197357177734375;-0.374292694368084710720978591780294664204120635986328125]
      mask Display: e = 0.06;c1 = [120 150 230]/255;c2 = ([120 150 230]+0)/383;c3 = ([120 150 230]+128)/383;patch([0 1 1 0],[0 0 1 1],c1);patch([0 1 1 1-e 1-e 0+e],[0 0 1 1-e 0+e 0+e],c2);patch([0 0 1 1-e 0+e 0+e],[0 1 1 1-e 1-e 0+e],c3);plot([0 1 1 0 0],[0 0 1 1 0]);disp('Weights');
  "IW{1,1}(54,:)'" : Constant  Value=[-0.2486484485608333738770880927404505200684070587158203125;0.83577728188382860441407729013008065521717071533203125;0.57486989095568052920981472198036499321460723876953125;0.97024081269379724989931901291129179298877716064453125;-0.98879255675692101501539355012937448918819427490234375;0.83912126110780660415144893704564310610294342041015625;0.11354912709266785919570708074388676322996616363525390625;-1.4348368794092400957396193916792981326580047607421875]
      mask Display: e = 0.06;c1 = [120 150 230]/255;c2 = ([120 150 230]+0)/383;c3 = ([120 150 230]+128)/383;patch([0 1 1 0],[0 0 1 1],c1);patch([0 1 1 1-e 1-e 0+e],[0 0 1 1-e 0+e 0+e],c2);patch([0 0 1 1-e 0+e 0+e],[0 1 1 1-e 1-e 0+e],c3);plot([0 1 1 0 0],[0 0 1 1 0]);disp('Weights');
  "IW{1,1}(55,:)'" : Constant  Value=[-1.3156402612456030709608967299573123455047607421875;-0.5652322322708627222453969807247631251811981201171875;0.08427929122864909194934313063640729524195194244384765625;-0.50910514221323055483736652604420669376850128173828125;1.2132629512387602677137010687147267162799835205078125;0.86491422656611394170766971001285128295421600341796875;1.086706505818441304000998570700176060199737548828125;-0.1678631890849177354940735540367313660681247711181640625]
      mask Display: e = 0.06;c1 = [120 150 230]/255;c2 = ([120 150 230]+0)/383;c3 = ([120 150 230]+128)/383;patch([0 1 1 0],[0 0 1 1],c1);patch([0 1 1 1-e 1-e 0+e],[0 0 1 1-e 0+e 0+e],c2);patch([0 0 1 1-e 0+e 0+e],[0 1 1 1-e 1-e 0+e],c3);plot([0 1 1 0 0],[0 0 1 1 0]);disp('Weights');
  "IW{1,1}(56,:)'" : Constant  Value=[-0.036958619579998595872094568903776234947144985198974609375;0.89138125115992494773564658316900022327899932861328125;0.31102308323696858938234299785108305513858795166015625;-1.2582495711248624647993210601271130144596099853515625;0.0345759870026162430267646641368628479540348052978515625;1.1449642712775729425089821233996190130710601806640625;0.9176626696629150981010525356396101415157318115234375;0.92631064719993883027626679904642514884471893310546875]
      mask Display: e = 0.06;c1 = [120 150 230]/255;c2 = ([120 150 230]+0)/383;c3 = ([120 150 230]+128)/383;patch([0 1 1 0],[0 0 1 1],c1);patch([0 1 1 1-e 1-e 0+e],[0 0 1 1-e 0+e 0+e],c2);patch([0 0 1 1-e 0+e 0+e],[0 1 1 1-e 1-e 0+e],c3);plot([0 1 1 0 0],[0 0 1 1 0]);disp('Weights');
  "IW{1,1}(57,:)'" : Constant  Value=[-1.00724358095364951992678470560349524021148681640625;-0.11423800723239700694033871286592329852283000946044921875;0.81762259902528011679123665089718997478485107421875;0.2385685609160678455342718962128856219351291656494140625;0.87400269509203354356685622406075708568096160888671875;1.0279933837142094521510671256692148745059967041015625;0.567795777674791946054710933822207152843475341796875;0.8792424542537933263020022423006594181060791015625]
      mask Display: e = 0.06;c1 = [120 150 230]/255;c2 = ([120 150 230]+0)/383;c3 = ([120 150 230]+128)/383;patch([0 1 1 0],[0 0 1 1],c1);patch([0 1 1 1-e 1-e 0+e],[0 0 1 1-e 0+e 0+e],c2);patch([0 0 1 1-e 0+e 0+e],[0 1 1 1-e 1-e 0+e],c3);plot([0 1 1 0 0],[0 0 1 1 0]);disp('Weights');
  "IW{1,1}(58,:)'" : Constant  Value=[0.7004698995780020975843171981978230178356170654296875;0.88657671142222016502643100466229952871799468994140625;0.25754513343583396167701948797912336885929107666015625;-1.0432939432904395626877658287412486970424652099609375;-0.69839431400561113871816587561625055968761444091796875;-1.0051011765149719945355855088564567267894744873046875;-1.0027198222317907916334434048621915280818939208984375;-0.1549416614681595749658526983694173395633697509765625]
      mask Display: e = 0.06;c1 = [120 150 230]/255;c2 = ([120 150 230]+0)/383;c3 = ([120 150 230]+128)/383;patch([0 1 1 0],[0 0 1 1],c1);patch([0 1 1 1-e 1-e 0+e],[0 0 1 1-e 0+e 0+e],c2);patch([0 0 1 1-e 0+e 0+e],[0 1 1 1-e 1-e 0+e],c3);plot([0 1 1 0 0],[0 0 1 1 0]);disp('Weights');
  "IW{1,1}(59,:)'" : Constant  Value=[-0.52249322809245146714829388656653463840484619140625;-0.038604714889007858691361008141029742546379566192626953125;0.9334425508727035580847086748690344393253326416015625;0.37118590673417017899993197715957649052143096923828125;-0.410784358150717732183210273433360271155834197998046875;1.2977180169749085170138869216316379606723785400390625;-0.84597439784161176934418335804366506636142730712890625;1.098884026551306902774740592576563358306884765625]
      mask Display: e = 0.06;c1 = [120 150 230]/255;c2 = ([120 150 230]+0)/383;c3 = ([120 150 230]+128)/383;patch([0 1 1 0],[0 0 1 1],c1);patch([0 1 1 1-e 1-e 0+e],[0 0 1 1-e 0+e 0+e],c2);patch([0 0 1 1-e 0+e 0+e],[0 1 1 1-e 1-e 0+e],c3);plot([0 1 1 0 0],[0 0 1 1 0]);disp('Weights');
  "IW{1,1}(6,:)'" : Constant  Value=[-0.2172824291542483077233072208400699310004711151123046875;-0.414389589626935450628053558830288238823413848876953125;-0.8756508556942150800495028306613676249980926513671875;-1.0700104105247232322284389738342724740505218505859375;0.433311908701625891904285481359693221747875213623046875;0.82413730567951148930916360768605954945087432861328125;-1.209111750613886204774871657718904316425323486328125;0.8394275694980957158719547805958427488803863525390625]
      mask Display: e = 0.06;c1 = [120 150 230]/255;c2 = ([120 150 230]+0)/383;c3 = ([120 150 230]+128)/383;patch([0 1 1 0],[0 0 1 1],c1);patch([0 1 1 1-e 1-e 0+e],[0 0 1 1-e 0+e 0+e],c2);patch([0 0 1 1-e 0+e 0+e],[0 1 1 1-e 1-e 0+e],c3);plot([0 1 1 0 0],[0 0 1 1 0]);disp('Weights');
  "IW{1,1}(60,:)'" : Constant  Value=[0.658035119967189441325672305538319051265716552734375;1.113031358541868964806553776725195348262786865234375;0.50542229864637244762803902631276287138462066650390625;0.81747877956618630879148668100242502987384796142578125;-1.3766929618750867181375951986410655081272125244140625;-0.50079045778376352071603605509153567254543304443359375;0.1760238701238831804385398527301731519401073455810546875;-0.459512398748305239681855027811252512037754058837890625]
      mask Display: e = 0.06;c1 = [120 150 230]/255;c2 = ([120 150 230]+0)/383;c3 = ([120 150 230]+128)/383;patch([0 1 1 0],[0 0 1 1],c1);patch([0 1 1 1-e 1-e 0+e],[0 0 1 1-e 0+e 0+e],c2);patch([0 0 1 1-e 0+e 0+e],[0 1 1 1-e 1-e 0+e],c3);plot([0 1 1 0 0],[0 0 1 1 0]);disp('Weights');
  "IW{1,1}(61,:)'" : Constant  Value=[0.392997873153709209592676643296726979315280914306640625;0.964888576391596419767893166863359510898590087890625;0.1732785805356214792194435858618817292153835296630859375;-0.245435378572325169077572581954882480204105377197265625;0.69999556142489149923591185142868198454380035400390625;-0.07631603231012946964018084372582961805164813995361328125;1.345729817646017512089429146726615726947784423828125;-1.1237471319022118709796131952316500246524810791015625]
      mask Display: e = 0.06;c1 = [120 150 230]/255;c2 = ([120 150 230]+0)/383;c3 = ([120 150 230]+128)/383;patch([0 1 1 0],[0 0 1 1],c1);patch([0 1 1 1-e 1-e 0+e],[0 0 1 1-e 0+e 0+e],c2);patch([0 0 1 1-e 0+e 0+e],[0 1 1 1-e 1-e 0+e],c3);plot([0 1 1 0 0],[0 0 1 1 0]);disp('Weights');
  "IW{1,1}(62,:)'" : Constant  Value=[1.301204190803214810756571750971488654613494873046875;-0.03582830036480200153192754441988654434680938720703125;-0.90118907558873961871626079300767742097377777099609375;0.3261562978140337687449346049106679856777191162109375;0.61034323081042851644184565884643234312534332275390625;-1.0011448909002655938138559577055275440216064453125;-1.183290887688753567630328689119778573513031005859375;0.364245021635683119409776509201037697494029998779296875]
      mask Display: e = 0.06;c1 = [120 150 230]/255;c2 = ([120 150 230]+0)/383;c3 = ([120 150 230]+128)/383;patch([0 1 1 0],[0 0 1 1],c1);patch([0 1 1 1-e 1-e 0+e],[0 0 1 1-e 0+e 0+e],c2);patch([0 0 1 1-e 0+e 0+e],[0 1 1 1-e 1-e 0+e],c3);plot([0 1 1 0 0],[0 0 1 1 0]);disp('Weights');
  "IW{1,1}(63,:)'" : Constant  Value=[-0.014413942292682946355597550791571848094463348388671875;0.5762056878721033559287434400175698101520538330078125;0.73889696621842626544918175568454898893833160400390625;0.71293275618026907824997806528699584305286407470703125;-0.7724211242051790549112411099486052989959716796875;1.3252669647170751687781375949271023273468017578125;0.886036386073798976070747812627814710140228271484375;0.197494150118838585061808998943888582289218902587890625]
      mask Display: e = 0.06;c1 = [120 150 230]/255;c2 = ([120 150 230]+0)/383;c3 = ([120 150 230]+128)/383;patch([0 1 1 0],[0 0 1 1],c1);patch([0 1 1 1-e 1-e 0+e],[0 0 1 1-e 0+e 0+e],c2);patch([0 0 1 1-e 0+e 0+e],[0 1 1 1-e 1-e 0+e],c3);plot([0 1 1 0 0],[0 0 1 1 0]);disp('Weights');
  "IW{1,1}(64,:)'" : Constant  Value=[-0.9509050009985642315513132416526786983013153076171875;0.1586148427159132789920903405800345353782176971435546875;0.1833392314949111590038910435396246612071990966796875;-0.3145089267586571590840094359009526669979095458984375;-1.893129491364980321321809242363087832927703857421875;-0.71082110101587991923821618911460973322391510009765625;-0.440796126378079911045659855517442338168621063232421875;-0.726888281546610670602603931911289691925048828125]
      mask Display: e = 0.06;c1 = [120 150 230]/255;c2 = ([120 150 230]+0)/383;c3 = ([120 150 230]+128)/383;patch([0 1 1 0],[0 0 1 1],c1);patch([0 1 1 1-e 1-e 0+e],[0 0 1 1-e 0+e 0+e],c2);patch([0 0 1 1-e 0+e 0+e],[0 1 1 1-e 1-e 0+e],c3);plot([0 1 1 0 0],[0 0 1 1 0]);disp('Weights');
  "IW{1,1}(7,:)'" : Constant  Value=[-0.105917907963459845266385173090384341776371002197265625;0.9950688560451304010001649658079259097576141357421875;0.667020016746283861408528537140227854251861572265625;1.158496743793929084631599835120141506195068359375;-0.213707519514648891512109685208997689187526702880859375;0.9040644041587257984105008290498517453670501708984375;-0.965974898104704937651376894791610538959503173828125;-0.89033961537106953709752588110859505832195281982421875]
      mask Display: e = 0.06;c1 = [120 150 230]/255;c2 = ([120 150 230]+0)/383;c3 = ([120 150 230]+128)/383;patch([0 1 1 0],[0 0 1 1],c1);patch([0 1 1 1-e 1-e 0+e],[0 0 1 1-e 0+e 0+e],c2);patch([0 0 1 1-e 0+e 0+e],[0 1 1 1-e 1-e 0+e],c3);plot([0 1 1 0 0],[0 0 1 1 0]);disp('Weights');
  "IW{1,1}(8,:)'" : Constant  Value=[-0.911660373731174811240407507284544408321380615234375;-0.70011210389034050916023943500476889312267303466796875;-0.6715163629904596920283665895112790167331695556640625;0.46878150580194988261695243636495433747768402099609375;-0.1281455115805487654512262452044524252414703369140625;0.565007414389368189944207188091240823268890380859375;0.40173886966572769363637007700162939727306365966796875;-1.65951097215210108259952903608791530132293701171875]
      mask Display: e = 0.06;c1 = [120 150 230]/255;c2 = ([120 150 230]+0)/383;c3 = ([120 150 230]+128)/383;patch([0 1 1 0],[0 0 1 1],c1);patch([0 1 1 1-e 1-e 0+e],[0 0 1 1-e 0+e 0+e],c2);patch([0 0 1 1-e 0+e 0+e],[0 1 1 1-e 1-e 0+e],c3);plot([0 1 1 0 0],[0 0 1 1 0]);disp('Weights');
  "IW{1,1}(9,:)'" : Constant  Value=[1.177033852232951094407553682685829699039459228515625;0.340050504893255556293496510988916270434856414794921875;-0.468007045946020550086785760868224315345287322998046875;1.1348829892461325119512594028492458164691925048828125;-0.08000522058520716239815584458483499474823474884033203125;0.494698360340561638093248575387406162917613983154296875;-1.08223086857544803507380493101663887500762939453125;-1.1599178929679399008279006011434830725193023681640625]
      mask Display: e = 0.06;c1 = [120 150 230]/255;c2 = ([120 150 230]+0)/383;c3 = ([120 150 230]+128)/383;patch([0 1 1 0],[0 0 1 1],c1);patch([0 1 1 1-e 1-e 0+e],[0 0 1 1-e 0+e 0+e],c2);patch([0 0 1 1-e 0+e 0+e],[0 1 1 1-e 1-e 0+e],c3);plot([0 1 1 0 0],[0 0 1 1 0]);disp('Weights');
  Mux : Mux  Inputs=64
      mask Display: e = 0.06;c1 = [120 150 230]/255;c2 = ([120 150 230]+0)/383;c3 = ([120 150 230]+128)/383;patch([0 1 1 0],[0 0 1 1],c1);patch([0 1 1 1-e 1-e 0+e],[0 0 1 1-e 0+e 0+e],c2);patch([0 0 1 1-e 0+e 0+e],[0 1 1 1-e 1-e 0+e],c3);plot([0 1 1 0 0],[0 0 1 1 0]);disp('Mux');
  dotprod{1..64} (64 alike) : neural/Weight Functions/dotprod
  "iz{1,1}" : Outport
      mask Display: e = 0.06;c1 = [120 230 180]/255;c2 = ([120 230 180]+0)/(256+128);c3 = ([120 230 180]+128)/(256+128);patch([0 1 1 0],[0 0 1 1],c1);patch([0 1 1 1-e 1-e 0+e],[0 0 1 1-e 0+e 0+e],c2);patch([0 0 1 1-e 0+e 0+e],[0 1 1 1-e 1-e 0+e],c3);plot([0 1 1 0 0],[0 0 1 1 0]);
  wires:
  "IW{1,1}(1,:)'"/1 -> dotprod1/1
  "pd{1,1}"/1 -> dotprod1/2, dotprod2/2, dotprod3/2, dotprod4/2, dotprod5/2, dotprod6/2, dotprod7/2, dotprod8/2, dotprod9/2, dotprod10/2, dotprod11/2, dotprod12/2, dotprod13/2, dotprod14/2, dotprod15/2, dotprod16/2, dotprod17/2, dotprod18/2, dotprod19/2, dotprod20/2, dotprod21/2, dotprod22/2, dotprod23/2, dotprod24/2, dotprod25/2, dotprod26/2, dotprod27/2, dotprod28/2, dotprod29/2, dotprod30/2, dotprod31/2, dotprod32/2, dotprod33/2, dotprod34/2, dotprod35/2, dotprod36/2, dotprod37/2, dotprod38/2, dotprod39/2, dotprod40/2, dotprod41/2, dotprod42/2, dotprod43/2, dotprod44/2, dotprod45/2, dotprod46/2, dotprod47/2, dotprod48/2, dotprod49/2, dotprod50/2, dotprod51/2, dotprod52/2, dotprod53/2, dotprod54/2, dotprod55/2, dotprod56/2, dotprod57/2, dotprod58/2, dotprod59/2, dotprod60/2, dotprod61/2, dotprod62/2, dotprod63/2, dotprod64/2
  dotprod1/1 -> Mux/1
  "IW{1,1}(2,:)'"/1 -> dotprod2/1
  dotprod2/1 -> Mux/2
  "IW{1,1}(3,:)'"/1 -> dotprod3/1
  dotprod3/1 -> Mux/3
  "IW{1,1}(4,:)'"/1 -> dotprod4/1
  dotprod4/1 -> Mux/4
  "IW{1,1}(5,:)'"/1 -> dotprod5/1
  dotprod5/1 -> Mux/5
  "IW{1,1}(6,:)'"/1 -> dotprod6/1
  dotprod6/1 -> Mux/6
  "IW{1,1}(7,:)'"/1 -> dotprod7/1
  dotprod7/1 -> Mux/7
  "IW{1,1}(8,:)'"/1 -> dotprod8/1
  dotprod8/1 -> Mux/8
  "IW{1,1}(9,:)'"/1 -> dotprod9/1
  dotprod9/1 -> Mux/9
  "IW{1,1}(10,:)'"/1 -> dotprod10/1
  dotprod10/1 -> Mux/10
  "IW{1,1}(11,:)'"/1 -> dotprod11/1
  dotprod11/1 -> Mux/11
  "IW{1,1}(12,:)'"/1 -> dotprod12/1
  dotprod12/1 -> Mux/12
  "IW{1,1}(13,:)'"/1 -> dotprod13/1
  dotprod13/1 -> Mux/13
  "IW{1,1}(14,:)'"/1 -> dotprod14/1
  dotprod14/1 -> Mux/14
  "IW{1,1}(15,:)'"/1 -> dotprod15/1
  dotprod15/1 -> Mux/15
  "IW{1,1}(16,:)'"/1 -> dotprod16/1
  dotprod16/1 -> Mux/16
  "IW{1,1}(17,:)'"/1 -> dotprod17/1
  dotprod17/1 -> Mux/17
  "IW{1,1}(18,:)'"/1 -> dotprod18/1
  dotprod18/1 -> Mux/18
  "IW{1,1}(19,:)'"/1 -> dotprod19/1
  dotprod19/1 -> Mux/19
  "IW{1,1}(20,:)'"/1 -> dotprod20/1
  dotprod20/1 -> Mux/20
  "IW{1,1}(21,:)'"/1 -> dotprod21/1
  dotprod21/1 -> Mux/21
  "IW{1,1}(22,:)'"/1 -> dotprod22/1
  dotprod22/1 -> Mux/22
  "IW{1,1}(23,:)'"/1 -> dotprod23/1
  dotprod23/1 -> Mux/23
  "IW{1,1}(24,:)'"/1 -> dotprod24/1
  dotprod24/1 -> Mux/24
  "IW{1,1}(25,:)'"/1 -> dotprod25/1
  dotprod25/1 -> Mux/25
  "IW{1,1}(26,:)'"/1 -> dotprod26/1
  dotprod26/1 -> Mux/26
  "IW{1,1}(27,:)'"/1 -> dotprod27/1
  dotprod27/1 -> Mux/27
  "IW{1,1}(28,:)'"/1 -> dotprod28/1
  dotprod28/1 -> Mux/28
  "IW{1,1}(29,:)'"/1 -> dotprod29/1
  dotprod29/1 -> Mux/29
  "IW{1,1}(30,:)'"/1 -> dotprod30/1
  dotprod30/1 -> Mux/30
  "IW{1,1}(31,:)'"/1 -> dotprod31/1
  dotprod31/1 -> Mux/31
  "IW{1,1}(32,:)'"/1 -> dotprod32/1
  dotprod32/1 -> Mux/32
  "IW{1,1}(33,:)'"/1 -> dotprod33/1
  dotprod33/1 -> Mux/33
  "IW{1,1}(34,:)'"/1 -> dotprod34/1
  dotprod34/1 -> Mux/34
  "IW{1,1}(35,:)'"/1 -> dotprod35/1
  dotprod35/1 -> Mux/35
  "IW{1,1}(36,:)'"/1 -> dotprod36/1
  dotprod36/1 -> Mux/36
  "IW{1,1}(37,:)'"/1 -> dotprod37/1
  dotprod37/1 -> Mux/37
  "IW{1,1}(38,:)'"/1 -> dotprod38/1
  dotprod38/1 -> Mux/38
  "IW{1,1}(39,:)'"/1 -> dotprod39/1
  dotprod39/1 -> Mux/39
  "IW{1,1}(40,:)'"/1 -> dotprod40/1
  dotprod40/1 -> Mux/40
  "IW{1,1}(41,:)'"/1 -> dotprod41/1
  dotprod41/1 -> Mux/41
  "IW{1,1}(42,:)'"/1 -> dotprod42/1
  dotprod42/1 -> Mux/42
  "IW{1,1}(43,:)'"/1 -> dotprod43/1
  dotprod43/1 -> Mux/43
  "IW{1,1}(44,:)'"/1 -> dotprod44/1
  dotprod44/1 -> Mux/44
  "IW{1,1}(45,:)'"/1 -> dotprod45/1
  dotprod45/1 -> Mux/45
  "IW{1,1}(46,:)'"/1 -> dotprod46/1
  dotprod46/1 -> Mux/46
  "IW{1,1}(47,:)'"/1 -> dotprod47/1
  dotprod47/1 -> Mux/47
  "IW{1,1}(48,:)'"/1 -> dotprod48/1
  dotprod48/1 -> Mux/48
  "IW{1,1}(49,:)'"/1 -> dotprod49/1
  dotprod49/1 -> Mux/49
  "IW{1,1}(50,:)'"/1 -> dotprod50/1
  dotprod50/1 -> Mux/50
  "IW{1,1}(51,:)'"/1 -> dotprod51/1
  dotprod51/1 -> Mux/51
  "IW{1,1}(52,:)'"/1 -> dotprod52/1
  dotprod52/1 -> Mux/52
  "IW{1,1}(53,:)'"/1 -> dotprod53/1
  dotprod53/1 -> Mux/53
  "IW{1,1}(54,:)'"/1 -> dotprod54/1
  dotprod54/1 -> Mux/54
  "IW{1,1}(55,:)'"/1 -> dotprod55/1
  dotprod55/1 -> Mux/55
  "IW{1,1}(56,:)'"/1 -> dotprod56/1
  dotprod56/1 -> Mux/56
  "IW{1,1}(57,:)'"/1 -> dotprod57/1
  dotprod57/1 -> Mux/57
  "IW{1,1}(58,:)'"/1 -> dotprod58/1
  dotprod58/1 -> Mux/58
  "IW{1,1}(59,:)'"/1 -> dotprod59/1
  dotprod59/1 -> Mux/59
  "IW{1,1}(60,:)'"/1 -> dotprod60/1
  dotprod60/1 -> Mux/60
  "IW{1,1}(61,:)'"/1 -> dotprod61/1
  dotprod61/1 -> Mux/61
  "IW{1,1}(62,:)'"/1 -> dotprod62/1
  dotprod62/1 -> Mux/62
  "IW{1,1}(63,:)'"/1 -> dotprod63/1
  dotprod63/1 -> Mux/63
  "IW{1,1}(64,:)'"/1 -> dotprod64/1
  dotprod64/1 -> Mux/64
  Mux/1 -> "iz{1,1}"/1
